simulink model "generic_20231123_1032"  (R2022b)
settings: Solver=ode45  StartTime=0.0  StopTime=50  RelTol=1e-3  EnableMultiTasking=on
model workspace (MAT data in the model file):
  A = 1
  Amplifier = -9.10007585438
  B = 1.19071237887
  K_d_yawrate = 0.231634180251
  K_dsteering = 5.24463953925
  k_speed = -0.570636497542
  k_stanley = 28.4909595466
  kd = -9.99955278144
  ki = 0.00519416981022
  kp = 9.99999979837
  path_curvature = 0
values from neighbouring files (symbols this model uses):
  brake_select = ones(length(speed), length(steering_angle))    [TwoDLook_uptable.m]
  curvature = 0.000:0.001:1    [TwoDLook_uptable.m]
  m = 1600    [MPCController1.m]    (also in MPCController2.m; MPC_Fmincon.m)
  speed = 0:0.1:100    [TwoDLook_uptable.m]
  steering_angle = -3.14/4:0.00628/4:3.14/4    [TwoDLook_uptable.m]
undefined symbols (not defined in the file or in its folder): DiscIntNeverNeededParam
libraries: CarMaker4SL x143, simulink x11, cstblocks x6, simulink_extras x4, autolibshared x1, mpcadaslib x1
(part 7 of 7)

== matlab function generic_20231123_1032/CarMaker/VehicleControl/CreateBus VhclCtrl/MPC_steering_controllers/Subsystem/MATLAB Function6 ==
  data: current_heading input; dt input; vx input; delta output; vy input
function delta = adaptive_steering_mpc(current_heading, dt, vx, vy)
    % Adaptive Model Predictive Controller (Adaptive MPC) for steering control
    persistent model_params theta
        
    function params = initialize_model_params(m, lf, lr, Iz)
        % Initialize model parameters
        % Define the state-space model
        A = [-2 * (lf + lr) / (m * vx), -vx - 2 * (lf * cf - lr * cr) / (m * vx);
             -2 * (lf * cf - lr * cr) / Iz, -2 * (lf^2 * cf + lr^2 * cr) / Iz];
    
        B = [2 * cf / m; 2 * lf * cf / Iz];
    
        % Store parameters in a struct
        params.A = A;
        params.B = B;
    end
    
    function dx = calculate_dynamics(u, params, vx, vy)
        % Calculate the dynamics of the system (Bicycle Model)
    
        % Unpack state variables
        vy1 = vy - params.B(2) * u;  % Correct lateral velocity for the tire slip angle
    
        % Bicycle model equations
        a = (2 * (u - vy1)) / (params.A(1, 2) * vx);
        b = (2 * lf * (u - vy1)) / params.A(2, 2);
    
        % State dynamics
        dx1 = a * dt;
        dx2 = b * dt;
    
        % Update state variables
        dx = [dx1; dx2];
    end

    % Define Q and R matrices
    Q = eye(2);  % Weighting matrix for state
    R = eye(1);  % Weighting matrix for control input

    % Define system parameters (replace these with your actual vehicle parameters)
    m = 1600;           % Vehicle mass [kg]
    l = 2.975;          % Wheelbase [m]
    Iz = 2986.624;      % Vehicle inertia [kg*m^2]
    cf = 80000;         % Front tire cornering stiffness [N/rad]
    cr = 120000;        % Rear tire cornering stiffness [N/rad]
    lf = 1.5;           % Distance from center of gravity to front axle [m]
    lr = 1.475;         % Distance from center of gravity to rear axle [m]

    % Adaptive parameters
    alpha = 0.1;  % Adaptation rate

    % Update the model parameters if not initialized
    if isempty(model_params)
        model_params = initialize_model_params(m, lf, lr, Iz);
    end

    % Update adaptive parameters if not initialized
    if isempty(theta)
        theta = [0.1; 0.1];  % Initial guess of parameters
    end

    % State vector (simplified, assuming current_heading is the heading error)
    x = [current_heading; 0];

    % Define matrices for quadprog
    H = blkdiag(Q, R);
    f = zeros(size(H, 1), 1);

    % Define linear inequality constraints for quadprog
    Aineq = [];
    Bineq = [];
    % Define linear equality constraints for quadprog
    Aeq = [];
    Beq = [];
    % Define lower and upper bounds for quadprog
    lb = [-1.6; -1.6; -1.6];  % Lower bounds on steering input for each dimension
    ub = [1.6; 1.6; 1.6];     % Upper bounds on steering input for each dimension


    % Initial guess for the control input
    u0 = zeros(size(H, 2), 1);  % Initialize u0 with the correct size

    % Solve the quadratic programming problem with quadprog
    options = optimoptions('quadprog', 'Display', 'off','Algorithm','active-set');
    [u_opt, ~, exitflag] = quadprog(H, f, Aineq, Bineq, Aeq, Beq, lb, ub, u0, options);

    % Check if optimization was successful
    if exitflag <= 0
        error('Quadprog failed to converge. Consider adjusting the problem formulation or solver options.');
    end

    % Update adaptive parameters online (using a simple gradient descent)
    %x_next = x + calculate_dynamics(u_opt, model_params, vx, vy);
    %theta = theta - alpha * (x_next - (x + calculate_dynamics(u_opt, model_params, vx, vy))) * x';

    % Extract control input (steering angle) from the optimization result
    delta = u_opt;
end

== matlab function generic_20231123_1032/CarMaker/VehicleControl/CreateBus VhclCtrl/MPC_steering_controllers/Subsystem/MATLAB Function7 ==
  data: u input; dt input; vx input; delta output; vy input; cr input; cf input; yaw input; dx output; dx1 output
function [delta,dx,dx1] = adaptive_steering_mpc(u, dt, vx, vy,cr,cf,yaw)
    % Adaptive Model Predictive Controller (Adaptive MPC) for steering control
   % persistent model_params theta
    % Define Q and R matrices
    Q = eye(2);  % Weighting matrix for state
    R = eye(1);  % Weighting matrix for control input

    % Define system parameters (replace these with your actual vehicle parameters)
    m = 1600;           % Vehicle mass [kg]
    l = 2.975;          % Wheelbase [m]
    Iz = 2986.624;      % Vehicle inertia [kg*m^2]
    %cf = 80000;         % Front tire cornering stiffness [N/rad]
    %cr = 120000;        % Rear tire cornering stiffness [N/rad]
    lf = 1.488;           % Distance from center of gravity to front axle [m]
    lr = -1.487;         % Distance from center of gravity to rear axle [m]
    if vx<0.5
        vx = 0.5;
    end
    function params = initialize_model_params(Iz,m,vx,cf,cr ,lf, lr)
        % Initialize model parameters
        % Define the state-space model
        A = [-(cr + cf) / (m * vx), -(lf * cf - lr * cr) / (m * vx)+vx^2;
             -(lf * cf - lr * cr) / (Iz*vx), -(lf^2 * cf + lr^2 * cr) / (Iz*vx)];
    
        B = [cf / m, cr/m; lf * cf / Iz, -lr*cr/Iz];
    
        % Store parameters in a struct
        params.A = A;
        params.B = B;
    end
    
    function [dx,dx1] = calculate_dynamics(params, yaw, vy,lf,dt,u)
        % Calculate the dynamics of the system (Bicycle Model)
    
        % Unpack state variables
        vy1 = vy - params.B(2) * u(1);  % Correct lateral velocity for the tire slip angle
        %vy1 = params.B(2);
        % Bicycle model equations
        %a = (2 * (u(1) - vy1)) / (params.A(1, 2) * vx);
        %b = (2 * lf * (u(2) - vy1)) / params.A(2, 2);
        % State dynamics
        %dx1 = a * dt;
        %dx2 = b * dt;
        dx1 = params.B *[0;u(2)]*dt;
        x_dot = params.A *[vy1;yaw]*dt+params.B *[0;u(2)]*dt;
        % Update state variables
        dx =x_dot; %[dx1; dx2];
    end
    params = initialize_model_params(Iz,m,vx,cf,cr ,lf, lr);
    [dx,dx1] = calculate_dynamics(params, yaw, vy,lf,dt,u);
    delta = atan(dx(2)*l/(vx*(1+ (-0.01*vx))));

%     % Adaptive parameters
%     alpha = 0.1;  % Adaptation rate
% 
%     % Update the model parameters if not initialized
%     if isempty(model_params)
%         model_params = initialize_model_params(m, lf, lr, Iz);
%     end
% 
%     % Update adaptive parameters if not initialized
%     if isempty(theta)
%         theta = [0.1; 0.1];  % Initial guess of parameters
%     end
% 
%     % State vector (simplified, assuming current_heading is the heading error)
%     x = [current_heading; 0];
% 
%     % Define matrices for quadprog
%     H = blkdiag(Q, R);
%     f = zeros(size(H, 1), 1);
% 
%     % Define linear inequality constraints for quadprog
%     Aineq = [];
%     Bineq = [];
%     % Define linear equality constraints for quadprog
%     Aeq = [];
%     Beq = [];
%     % Define lower and upper bounds for quadprog
%     lb = [-1.6; -1.6; -1.6];  % Lower bounds on steering input for each dimension
%     ub = [1.6; 1.6; 1.6];     % Upper bounds on steering input for each dimension
% 
% 
%     % Initial guess for the control input
%     u0 = zeros(size(H, 2), 1);  % Initialize u0 with the correct size
% 
%     % Solve the quadratic programming problem with quadprog
%     options = optimoptions('quadprog', 'Display', 'off','Algorithm','active-set');
%     [u_opt, ~, exitflag] = quadprog(H, f, Aineq, Bineq, Aeq, Beq, lb, ub, u0, options);
% 
%     % Check if optimization was successful
%     if exitflag <= 0
%         error('Quadprog failed to converge. Consider adjusting the problem formulation or solver options.');
%     end
% 
%     % Update adaptive parameters online (using a simple gradient descent)
%     %x_next = x + calculate_dynamics(u_opt, model_params, vx, vy);
%     %theta = theta - alpha * (x_next - (x + calculate_dynamics(u_opt, model_params, vx, vy))) * x';
% 
%     % Extract control input (steering angle) from the optimization result
%     delta = u_opt;
end

== matlab function generic_20231123_1032/CarMaker/VehicleControl/CreateBus VhclCtrl/MPC_steering_controllers/Traditional_MPC/MPC_steering_control ==
  data: Lateral_deviation input; steering_cmd output; A input; B input
function steering_cmd = MPC_Steering_control(Lateral_deviation,A,B)
    % Model Predictive Controller (MPC) for speed contol
    %speed_ref  = speed_rf+0.4;
    %Lateral_deviation= current_speed - speed_ref;
    % Define MPC parameters
    Ts = 0.1;  % Sampling time
    N = 10;    % Prediction horizon
    Q = 1;     % State weight
    R = 1;     % Input weight
    S = 0.1;   % Terminal state weight (integral term)
    
    % State-space model (simplified for illustration)
    %A = 0.8;
    %B = Ts;
    
    % Define cost and constraints for fmincon
    costFunction = @(u) (Lateral_deviation + B * u)' * Q * (Lateral_deviation + B * u) + u' * R * u + S * sum(u);
    Aeq = [];
    Beq = [];
    Aineq = [];
    Bineq = [];
    lb = -1.6; % Lower bound on throttle_Brake
    ub = 1.6;  % Upper bound on throttle_Brake
    
    % Steady-state error constraint
    Aineq = [Aineq; B];
    Bineq = [Bineq; -Lateral_deviation];
    
    % Initial guess
    u0 = 0;
    
    % Solve optimization problem
    options = optimoptions('fmincon', 'Display', 'off', 'Algorithm', 'sqp');
    u_opt = fmincon(costFunction, u0, Aineq, Bineq, Aeq, Beq, lb, ub, [], options);
    
    % Extract control input (throttle_Brake) from the optimization result
    steering_cmd = u_opt;
end

== matlab function generic_20231123_1032/CarMaker/VehicleControl/CreateBus VhclCtrl/MPC_steering_controllers/Traditional_MPC/MPC_steering_control1 ==
  data: Heading_error input; steering_cmd output; A input; B input
function steering_cmd = MPC_Steering_control(Heading_error,A,B)
    % Model Predictive Controller (MPC) for speed contol
    %speed_ref  = speed_rf+0.4;
    %Heading_error= current_speed - speed_ref;
    % Define MPC parameters
    Ts = 0.1;  % Sampling time
    N = 10;    % Prediction horizon
    Q = 1;     % State weight
    R = 1;     % Input weight
    S = 0.1;   % Terminal state weight (integral term)
    
    % State-space model (simplified for illustration)
    %A = 0.8;
    %B = Ts;
    
    % Define cost and constraints for fmincon
    costFunction = @(u) (Heading_error + B * u)' * Q * (Heading_error + B * u) + u' * R * u + S * sum(u);
    Aeq = [];
    Beq = [];
    Aineq = [];
    Bineq = [];
    lb = -1.6; % Lower bound on throttle_Brake
    ub = 1.6;  % Upper bound on throttle_Brake
    
    % Steady-state error constraint
    Aineq = [Aineq; B];
    Bineq = [Bineq; -Heading_error];
    
    % Initial guess
    u0 = 0;
    
    % Solve optimization problem
    options = optimoptions('fmincon', 'Display', 'off', 'Algorithm', 'sqp');
    u_opt = fmincon(costFunction, u0, Aineq, Bineq, Aeq, Beq, lb, ub, [], options);
    
    % Extract control input (throttle_Brake) from the optimization result
    steering_cmd = u_opt;
end

== matlab function generic_20231123_1032/CarMaker/VehicleControl/CreateBus VhclCtrl.Steering/MATLAB Function2 ==
  data: x_car input; nw_pth_gtd output; y_car input; trgt_x input; trgt_y input
function nw_pth_gtd = fcn(x_car,y_car,trgt_x,trgt_y)
nw_pth_gtd = zeros(2,1);
nw_pth_gtd(1,1) = x_car+trgt_x;
nw_pth_gtd(2,1) = y_car + trgt_y;

== matlab function generic_20231123_1032/CarMaker/VehicleControl/CreateBus VhclCtrl/Stanley steering & speed//Brake controller/Stanley_controller_with_thottle_and_brake_commands/MPCLongitudianl_contorl/MPC_speed_control ==
  data: speed_error input; throttle_Brake output; A input; B input
function throttle_Brake = MPC_speed_control(speed_error,A,B)
    % Model Predictive Controller (MPC) for speed contol
    %speed_ref  = speed_rf+0.4;
    %speed_error= current_speed - speed_ref;
    % Define MPC parameters
    Ts = 0.1;  % Sampling time
    N = 10;    % Prediction horizon
    Q = 1;     % State weight
    R = 1;     % Input weight
    S = 0.1;   % Terminal state weight (integral term)
    
    % State-space model (simplified for illustration)
    %A = 0.8;
    %B = Ts;
    
    % Define cost and constraints for fmincon
    costFunction = @(u) (speed_error + B * u)' * Q * (speed_error + B * u) + u' * R * u + S * sum(u);
    Aeq = [];
    Beq = [];
    Aineq = [];
    Bineq = [];
    lb = 0; % Lower bound on throttle_Brake
    ub = 1;  % Upper bound on throttle_Brake
    
    % Steady-state error constraint
    Aineq = [Aineq; B];
    Bineq = [Bineq; -speed_error];
    
    % Initial guess
    u0 = 0;
    
    % Solve optimization problem
    options = optimoptions('fmincon', 'Display', 'off', 'Algorithm', 'sqp');
    u_opt = fmincon(costFunction, u0, Aineq, Bineq, Aeq, Beq, lb, ub, [], options);
    
    % Extract control input (throttle_Brake) from the optimization result
    throttle_Brake = u_opt;
end

== matlab function generic_20231123_1032/CarMaker/VehicleControl/Subsystem1/Cross_track_error_calcuation/Cross_track_error_calcuation ==
  data: x_vehicle input; cte output; y_vehicle input; x_point input; y_point input; denominator output; x2 input; y2 input
function [cte,denominator]= calculate_cross_track_error(x_vehicle, y_vehicle, x_point, y_point,x2,y2)
    % Calculate cross-track error for a given vehicle position and single point
    function cte = calculate_perpendicular_distance(x_vehicle, y_vehicle, x_point, y_point)
    % Calculate the perpendicular distance from the vehicle to the point

    % Coordinates of the point
    x1 = x_point;
    y1 = y_point;
    %x2 = x_vehicle;
    %y2 = y_vehicle;

    % Calculate the cross-track error using the formula for the distance from a point to a line
    numerator = (x2 - x1) * (y1 - y_vehicle) - (x1 - x_vehicle) * (y2 - y1);
    denominator = sqrt((x2 - x1)^2 + (y2 - y1)^2);

    % Ensure that the denominator is not zero to avoid division by zero
    if denominator ~= 0
        cte = (numerator / denominator);
    else
        cte = 0;
    end
end
    % Calculate cross-track error as the perpendicular distance
    cte = calculate_perpendicular_distance(x_vehicle, y_vehicle, x_point, y_point);
end

== matlab function generic_20231123_1032/CarMaker/VehicleControl/Subsystem1/calculate_cross_track_error/calculate_cross_track_error ==
  data: x_vehicle input; cte output; y_vehicle input; x_point input; y_point input; slope output; x2 input; y2 input
function [cte,slope]= calculate_cross_track_error(x_vehicle, y_vehicle, x_point, y_point,x2,y2)
    % Calculate cross-track error for a given vehicle position and single point
    function cte = calculate_perpendicular_distance(x_vehicle, y_vehicle, x_point, y_point)
    % Calculate the perpendicular distance from the vehicle to the point

    % Coordinates of the point
    x1 = x_point;
    y1 = y_point;
    %x2 = x_vehicle;
    %y2 = y_vehicle;
    slope =  atan((y2-y1)/(x2-x1));
    % Calculate the cross-track error using the formula for the distance from a point to a line
    numerator = (x2 - x1) * (y1 - y_vehicle) - (x1 - x_vehicle) * (y2 - y1);
    denominator = sqrt((x2 - x1)^2 + (y2 - y1)^2);

    % Ensure that the denominator is not zero to avoid division by zero
    if denominator ~= 0
        cte = (numerator / denominator);
    else
        cte = 0;
    end
end
    % Calculate cross-track error as the perpendicular distance
    cte = calculate_perpendicular_distance(x_vehicle, y_vehicle, x_point, y_point);
end
